simulink model "parte2"  (R2022b)
settings: Solver=VariableStepAuto  StartTime=0.0  StopTime=10/60  RelTol=1e-3
libraries: spsSeriesRLCBranchLib x9, spsFourierLib x6, spsACVoltageSourceLib x6, spsGroundLib x3, spsCurrentMeasurementLib x3, spsVoltageMeasurementLib x3, spsThreePhaseVIMeasurementLib x2, spsThreePhaseProgrammableVoltageSourceLib x1, sps_lib x1
settings Model: Creator=mateo  LastModifiedBy=mateo

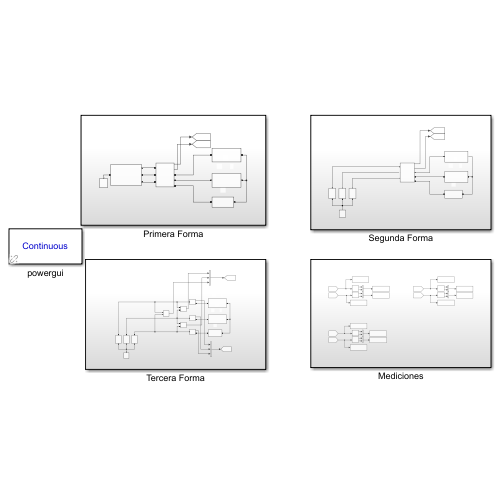
[thumbnail: Simulink's stored preview of the top-level diagram]
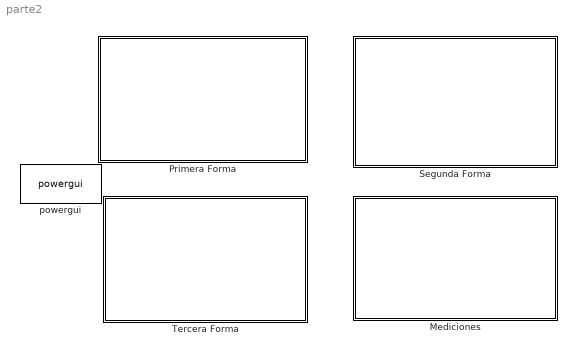
== system parte2 ==
  Mediciones : Subsystem
  Primera Forma : Subsystem
  Segunda Forma : Subsystem
  Tercera Forma : Subsystem
  powergui : sps_lib/powergui  Priority=1  SimulationMode=Continuous  SampleTime=50e-6  frequency=60  Iterations=50  frequencyindice=60  Pbase=100e6  ErrMax=1e-4  UnitsV=kV  UnitsW=MW  buscounter=0  FunctionMessages=off  echomessages=off  EnableUseOfTLC=off  CurrentSourceSwitches=off  DisableSnubberDevices=off  DisableRonSwitches=off  DisableVfSwitches=off  DisplayEquations=off  AutomaticDiscreteSolvers=off  SolverType=Tustin/Backward Euler (TBE)  Interpol=off  ExternalGateDelay=off  methode=off  Ts=100  x0status=blocks  SPID=on  SwTol=0  HookPort=off  NonlinearTolerance=1e-4  nMaxIteration=100  ContinueOnMaxIteration=off  RestoreLinks=warning  ResistiveCurrentMeasurement=off  Frange=[0:2:500]  Ylog=off  Xlog=on  ShowGrid=off  save=off  variable=ZData  structure=0  ZoomFFT=off  StartTime=0.0  cycles=1  DisplayStyle=1  fundamental=60  FreqAxis=off  MaxFrequency=1000  frequencyindicesteady=1  RmsSteady=1  display=off

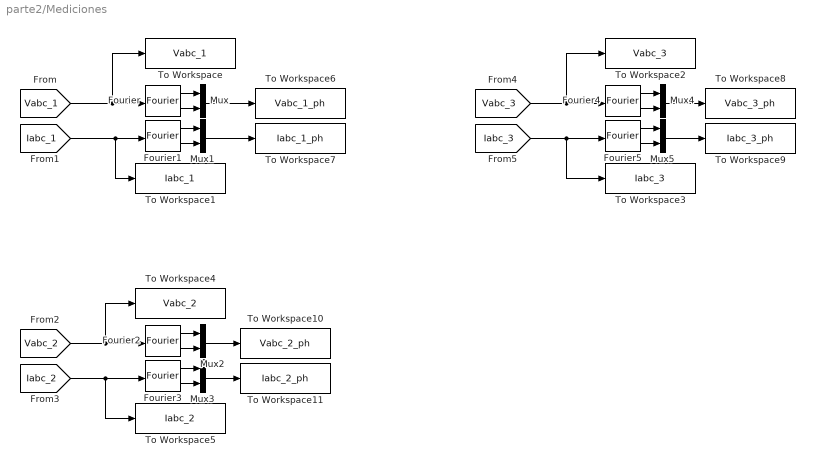
== system parte2/Mediciones ==
  Fourier{,1..5} (6 alike) : spsFourierLib/Fourier  Freq=60  n=1  InInit=[0, 0]  Ts=0
  Mux{,1..5} (6 alike) : Mux  Inputs=2
  To Workspace : ToWorkspace  VariableName=Vabc_1  SaveFormat=Timeseries  SampleTime=-1
  To Workspace1 : ToWorkspace  VariableName=Iabc_1  SaveFormat=Timeseries  SampleTime=-1
  To Workspace10 : ToWorkspace  VariableName=Vabc_2_ph  SaveFormat=Timeseries  SampleTime=-1
  To Workspace11 : ToWorkspace  VariableName=Iabc_2_ph  SaveFormat=Timeseries  SampleTime=-1
  To Workspace2 : ToWorkspace  VariableName=Vabc_3  SaveFormat=Timeseries  SampleTime=-1
  To Workspace3 : ToWorkspace  VariableName=Iabc_3  SaveFormat=Timeseries  SampleTime=-1
  To Workspace4 : ToWorkspace  VariableName=Vabc_2  SaveFormat=Timeseries  SampleTime=-1
  To Workspace5 : ToWorkspace  VariableName=Iabc_2  SaveFormat=Timeseries  SampleTime=-1
  To Workspace6 : ToWorkspace  VariableName=Vabc_1_ph  SaveFormat=Timeseries  SampleTime=-1
  To Workspace7 : ToWorkspace  VariableName=Iabc_1_ph  SaveFormat=Timeseries  SampleTime=-1
  To Workspace8 : ToWorkspace  VariableName=Vabc_3_ph  SaveFormat=Timeseries  SampleTime=-1
  To Workspace9 : ToWorkspace  VariableName=Iabc_3_ph  SaveFormat=Timeseries  SampleTime=-1
  wires:
  [Vabc_1] -> To Workspace/1, Fourier/1
  [Iabc_1] -> To Workspace1/1, Fourier1/1
  [Vabc_2] -> To Workspace4/1, Fourier2/1
  [Iabc_2] -> To Workspace5/1, Fourier3/1
  [Vabc_3] -> To Workspace2/1, Fourier4/1
  [Iabc_3] -> To Workspace3/1, Fourier5/1
  Fourier/1 -> Mux/1
  Fourier/2 -> Mux/2
  Fourier1/2 -> Mux1/2
  Fourier1/1 -> Mux1/1
  Fourier2/1 -> Mux2/1
  Fourier2/2 -> Mux2/2
  Fourier3/2 -> Mux3/2
  Fourier3/1 -> Mux3/1
  Fourier4/1 -> Mux4/1
  Fourier4/2 -> Mux4/2
  Fourier5/1 -> Mux5/1
  Fourier5/2 -> Mux5/2
  Mux/1 -> To Workspace6/1
  Mux1/1 -> To Workspace7/1
  Mux3/1 -> To Workspace11/1
  Mux2/1 -> To Workspace10/1
  Mux5/1 -> To Workspace9/1
  Mux4/1 -> To Workspace8/1

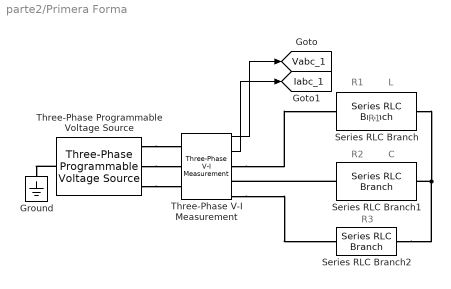
== system parte2/Primera Forma ==
  note: R1
  note: R1
  note: L
  note: R2
  note: C
  note: R3
  Ground : spsGroundLib/Ground  LConnTagsString=a
  Series RLC Branch : spsSeriesRLCBranchLib/Series RLC Branch  LConnTagsString=__new0  RConnTagsString=__new0  BranchType=RL  Resistance=250  Inductance=160e-3  SetiL0=off  InitialCurrent=0  Capacitance=1e-6  Setx0=off  InitialVoltage=0  Measurements=None
  Series RLC Branch1 : spsSeriesRLCBranchLib/Series RLC Branch  LConnTagsString=__new0  RConnTagsString=__new0  BranchType=RC  Resistance=320  Inductance=160e-3  SetiL0=off  InitialCurrent=0  Capacitance=22e-6  Setx0=off  InitialVoltage=0  Measurements=None
  Series RLC Branch2 : spsSeriesRLCBranchLib/Series RLC Branch  LConnTagsString=__new0  RConnTagsString=__new0  BranchType=R  Resistance=330  Inductance=160e-3  SetiL0=off  InitialCurrent=0  Capacitance=1e-6  Setx0=off  InitialVoltage=0  Measurements=None
  Three-Phase Programmable Voltage Source : spsThreePhaseProgrammableVoltageSourceLib/Three-Phase Programmable Voltage Source  PositiveSequence="[215  0 60]"  VariationEntity=None  VariationType=Table of time-amplitude pairs  VariationTypeAlt=Step  VariationStep=0.5  VariationRate=10  VariationMagnitude=0.3  VariationFrequency=2  VariationTiming=[1 2]  VariationPhaseA=off  Amplitudes=[1 0.8 1.2 1.0]  TimeValues=[0 0.1 0.15 0.2]  HarmonicGeneration=off  HarmonicA=[3 0.2 -25 0]  HarmonicB=[2 0.15 35 2]  Timing="[0.05  3]"  BusType=swing  Pref=0  Qref=0  Qmin=-inf  Qmax=inf
  Three-Phase V-I Measurement : spsThreePhaseVIMeasurementLib/Three-Phase V-I Measurement  VoltageMeasurement=phase-to-phase  SetLabelV=off  LabelV=Vabc  Vpu=off  VpuLL=off  CurrentMeasurement=yes  SetLabelI=off  LabelI=Iabc  Ipu=off  Pbase=100e6  Vbase=500e3  OutputType=Complex  PhasorSimulation=off  PSBequivalent=0
  tag scope: Iabc_1=global, Vabc_1=global
  wires:
  Three-Phase V-I Measurement/1 -> [Vabc_1]
  Three-Phase V-I Measurement/2 -> [Iabc_1]
  connections:
  Three-Phase V-I Measurement/RConn3 -- Series RLC Branch2/LConn1
  Three-Phase Programmable Voltage Source/RConn3 -- Three-Phase V-I Measurement/LConn3
  Series RLC Branch1/LConn1 -- Three-Phase V-I Measurement/RConn2
  Three-Phase Programmable Voltage Source/LConn1 -- Ground/LConn1
  Series RLC Branch/RConn1 -- Series RLC Branch2/RConn1 -- Series RLC Branch1/RConn1
  Three-Phase Programmable Voltage Source/RConn2 -- Three-Phase V-I Measurement/LConn2
  Three-Phase V-I Measurement/RConn1 -- Series RLC Branch/LConn1
  Three-Phase Programmable Voltage Source/RConn1 -- Three-Phase V-I Measurement/LConn1

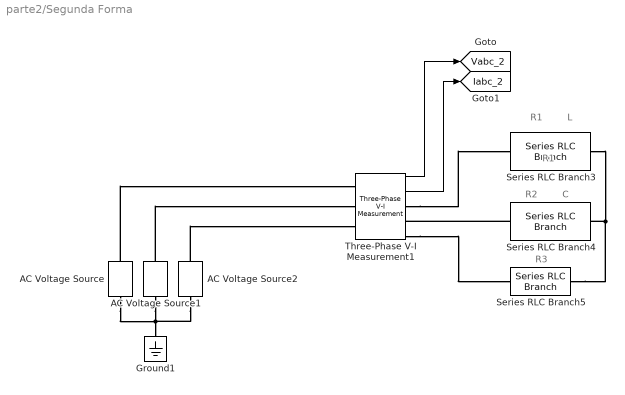
== system parte2/Segunda Forma ==
  note: C
  note: R2
  note: L
  note: R1
  note: R3
  note: R1
  AC Voltage Source : spsACVoltageSourceLib/AC Voltage Source  Amplitude=sqrt(2)*215/sqrt(3)  Phase=0  Frequency=60  SampleTime=0  Measurements=None  BusType=swing  Pref=10e3  Qref=0  Qmin=-inf  Qmax=+inf
  AC Voltage Source1 : spsACVoltageSourceLib/AC Voltage Source  Amplitude=sqrt(2)*215/sqrt(3)  Phase=-120  Frequency=60  SampleTime=0  Measurements=None  BusType=swing  Pref=10e3  Qref=0  Qmin=-inf  Qmax=+inf
  AC Voltage Source2 : spsACVoltageSourceLib/AC Voltage Source  Amplitude=sqrt(2)*215/sqrt(3)  Phase=120  Frequency=60  SampleTime=0  Measurements=None  BusType=swing  Pref=10e3  Qref=0  Qmin=-inf  Qmax=+inf
  Ground1 : spsGroundLib/Ground  LConnTagsString=a
  Series RLC Branch3 : spsSeriesRLCBranchLib/Series RLC Branch  LConnTagsString=__new0  RConnTagsString=__new0  BranchType=RL  Resistance=250  Inductance=160e-3  SetiL0=off  InitialCurrent=0  Capacitance=1e-6  Setx0=off  InitialVoltage=0  Measurements=None
  Series RLC Branch4 : spsSeriesRLCBranchLib/Series RLC Branch  LConnTagsString=__new0  RConnTagsString=__new0  BranchType=RC  Resistance=320  Inductance=160e-3  SetiL0=off  InitialCurrent=0  Capacitance=22e-6  Setx0=off  InitialVoltage=0  Measurements=None
  Series RLC Branch5 : spsSeriesRLCBranchLib/Series RLC Branch  LConnTagsString=__new0  RConnTagsString=__new0  BranchType=R  Resistance=330  Inductance=160e-3  SetiL0=off  InitialCurrent=0  Capacitance=1e-6  Setx0=off  InitialVoltage=0  Measurements=None
  Three-Phase V-I Measurement1 : spsThreePhaseVIMeasurementLib/Three-Phase V-I Measurement  VoltageMeasurement=phase-to-phase  SetLabelV=off  LabelV=Vabc  Vpu=off  VpuLL=off  CurrentMeasurement=yes  SetLabelI=off  LabelI=Iabc  Ipu=off  Pbase=100e6  Vbase=500e3  OutputType=Complex  PhasorSimulation=off  PSBequivalent=0
  tag scope: Iabc_2=global, Vabc_2=global
  wires:
  Three-Phase V-I Measurement1/2 -> [Iabc_2]
  Three-Phase V-I Measurement1/1 -> [Vabc_2]
  connections:
  AC Voltage Source2/LConn1 -- AC Voltage Source/LConn1 -- AC Voltage Source1/LConn1 -- Ground1/LConn1
  Series RLC Branch4/RConn1 -- Series RLC Branch3/RConn1 -- Series RLC Branch5/RConn1
  Three-Phase V-I Measurement1/RConn3 -- Series RLC Branch5/LConn1
  Series RLC Branch4/LConn1 -- Three-Phase V-I Measurement1/RConn2
  AC Voltage Source1/RConn1 -- Three-Phase V-I Measurement1/LConn2
  Three-Phase V-I Measurement1/RConn1 -- Series RLC Branch3/LConn1
  AC Voltage Source2/RConn1 -- Three-Phase V-I Measurement1/LConn3
  AC Voltage Source/RConn1 -- Three-Phase V-I Measurement1/LConn1

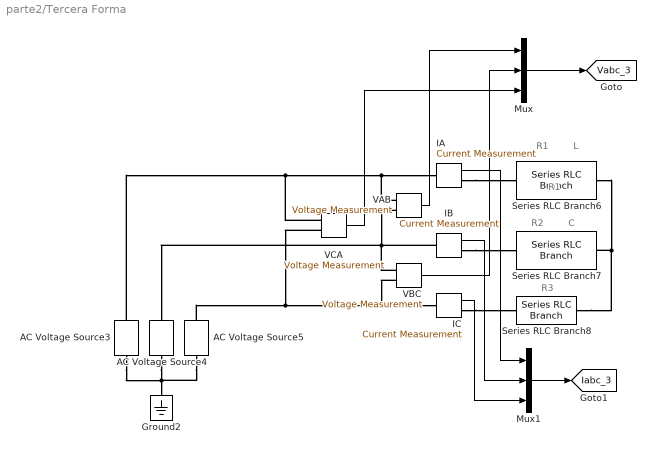
== system parte2/Tercera Forma ==
  note: R3
  note: R1
  note: R2
  note: C
  note: R1
  note: L
  AC Voltage Source3 : spsACVoltageSourceLib/AC Voltage Source  Amplitude=sqrt(2)*215/sqrt(3)  Phase=0  Frequency=60  SampleTime=0  Measurements=None  BusType=swing  Pref=10e3  Qref=0  Qmin=-inf  Qmax=+inf
  AC Voltage Source4 : spsACVoltageSourceLib/AC Voltage Source  Amplitude=sqrt(2)*215/sqrt(3)  Phase=-120  Frequency=60  SampleTime=0  Measurements=None  BusType=swing  Pref=10e3  Qref=0  Qmin=-inf  Qmax=+inf
  AC Voltage Source5 : spsACVoltageSourceLib/AC Voltage Source  Amplitude=sqrt(2)*215/sqrt(3)  Phase=120  Frequency=60  SampleTime=0  Measurements=None  BusType=swing  Pref=10e3  Qref=0  Qmin=-inf  Qmax=+inf
  Ground2 : spsGroundLib/Ground  LConnTagsString=a
  IA : spsCurrentMeasurementLib/Current Measurement  PhasorSimulation=off  OutputType=Complex  PSBequivalent=0
  IB : spsCurrentMeasurementLib/Current Measurement  PhasorSimulation=off  OutputType=Complex  PSBequivalent=0
  IC : spsCurrentMeasurementLib/Current Measurement  PhasorSimulation=off  OutputType=Complex  PSBequivalent=0
  Mux : Mux  Inputs=3
  Mux1 : Mux  Inputs=3
  Series RLC Branch6 : spsSeriesRLCBranchLib/Series RLC Branch  LConnTagsString=__new0  RConnTagsString=__new0  BranchType=RL  Resistance=250  Inductance=160e-3  SetiL0=off  InitialCurrent=0  Capacitance=1e-6  Setx0=off  InitialVoltage=0  Measurements=None
  Series RLC Branch7 : spsSeriesRLCBranchLib/Series RLC Branch  LConnTagsString=__new0  RConnTagsString=__new0  BranchType=RC  Resistance=320  Inductance=160e-3  SetiL0=off  InitialCurrent=0  Capacitance=22e-6  Setx0=off  InitialVoltage=0  Measurements=None
  Series RLC Branch8 : spsSeriesRLCBranchLib/Series RLC Branch  LConnTagsString=__new0  RConnTagsString=__new0  BranchType=R  Resistance=330  Inductance=160e-3  SetiL0=off  InitialCurrent=0  Capacitance=1e-6  Setx0=off  InitialVoltage=0  Measurements=None
  VAB : spsVoltageMeasurementLib/Voltage Measurement  PhasorSimulation=off  OutputType=Complex  PSBequivalent=0
  VBC : spsVoltageMeasurementLib/Voltage Measurement  PhasorSimulation=off  OutputType=Complex  PSBequivalent=0
  VCA : spsVoltageMeasurementLib/Voltage Measurement  PhasorSimulation=off  OutputType=Complex  PSBequivalent=0
  tag scope: Iabc_3=global, Vabc_3=global
  wires:
  VAB/1 -> Mux/1
  VBC/1 -> Mux/2
  VCA/1 -> Mux/3
  IA/1 -> Mux1/1
  IB/1 -> Mux1/2
  IC/1 -> Mux1/3
  Mux/1 -> [Vabc_3]
  Mux1/1 -> [Iabc_3]
  connections:
  IC/RConn1 -- Series RLC Branch8/LConn1
  Series RLC Branch8/RConn1 -- Series RLC Branch7/RConn1 -- Series RLC Branch6/RConn1
  AC Voltage Source5/LConn1 -- AC Voltage Source3/LConn1 -- AC Voltage Source4/LConn1 -- Ground2/LConn1
  IB/LConn1 -- AC Voltage Source4/RConn1 -- VBC/LConn1 -- VAB/LConn2
  AC Voltage Source5/RConn1 -- VCA/LConn1 -- VBC/LConn2 -- IC/LConn1
  AC Voltage Source3/RConn1 -- VCA/LConn2 -- VAB/LConn1 -- IA/LConn1
  IB/RConn1 -- Series RLC Branch7/LConn1
  IA/RConn1 -- Series RLC Branch6/LConn1
